simulink library "MBDS_Subsystems"  (R2018b)
settings: Solver=ode45  StartTime=0.0  StopTime=10.0  RelTol=1e-3
libraries: KIBES_Signal x1429, MBDS_Modules x44, simulink x2
(part 4 of 15)

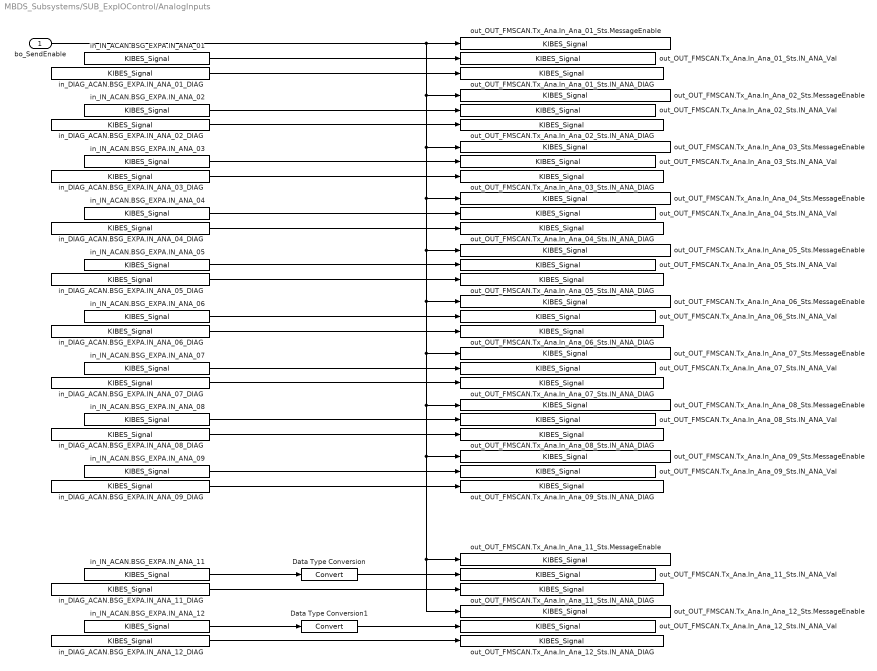
== system MBDS_Subsystems/SUB_ExpIOControl/AnalogInputs ==
  bo_SendEnable : Inport
  Data Type Conversion : DataTypeConversion  InitFcn=|  SaturateOnIntegerOverflow=on
      | try
      |    MBDS_BlockCallback('Update', gcb);
      | end
      settings: AttributesFormatString=Saturate: %<SaturateOnIntegerOverflow>
  Data Type Conversion1 : DataTypeConversion  InitFcn=|  SaturateOnIntegerOverflow=on
      | try
      |    MBDS_BlockCallback('Update', gcb);
      | end
      settings: AttributesFormatString=Saturate: %<SaturateOnIntegerOverflow>
  in_DIAG_ACAN.BSG_EXPA.IN_ANA_01_DIAG : KIBES_Signal/KIBES_Signal  MBDS_LibraryBlock=on  DatabaseKey=815  SignalName=DIAG_ACAN.BSG_EXPA.IN_ANA_01_DIAG  SymbolName=DIAG_ACAN_BSG_EXPA_IN_ANA_01_DIAG_000815  DataType=uint16  Init=1  Slope=1  Bias=0  DataSize=1  fpDataType=uint16  BlockIOType=Inport  DeviceType=0
  in_DIAG_ACAN.BSG_EXPA.IN_ANA_02_DIAG : KIBES_Signal/KIBES_Signal  MBDS_LibraryBlock=on  DatabaseKey=819  SignalName=DIAG_ACAN.BSG_EXPA.IN_ANA_02_DIAG  SymbolName=DIAG_ACAN_BSG_EXPA_IN_ANA_02_DIAG_000819  DataType=uint16  Init=1  Slope=1  Bias=0  DataSize=1  fpDataType=uint16  BlockIOType=Inport  DeviceType=0
  in_DIAG_ACAN.BSG_EXPA.IN_ANA_03_DIAG : KIBES_Signal/KIBES_Signal  MBDS_LibraryBlock=on  DatabaseKey=822  SignalName=DIAG_ACAN.BSG_EXPA.IN_ANA_03_DIAG  SymbolName=DIAG_ACAN_BSG_EXPA_IN_ANA_03_DIAG_000822  DataType=uint16  Init=1  Slope=1  Bias=0  DataSize=1  fpDataType=uint16  BlockIOType=Inport  DeviceType=0
  in_DIAG_ACAN.BSG_EXPA.IN_ANA_04_DIAG : KIBES_Signal/KIBES_Signal  MBDS_LibraryBlock=on  DatabaseKey=824  SignalName=DIAG_ACAN.BSG_EXPA.IN_ANA_04_DIAG  SymbolName=DIAG_ACAN_BSG_EXPA_IN_ANA_04_DIAG_000824  DataType=uint16  Init=1  Slope=1  Bias=0  DataSize=1  fpDataType=uint16  BlockIOType=Inport  DeviceType=0
  in_DIAG_ACAN.BSG_EXPA.IN_ANA_05_DIAG : KIBES_Signal/KIBES_Signal  MBDS_LibraryBlock=on  DatabaseKey=826  SignalName=DIAG_ACAN.BSG_EXPA.IN_ANA_05_DIAG  SymbolName=DIAG_ACAN_BSG_EXPA_IN_ANA_05_DIAG_000826  DataType=uint16  Init=1  Slope=1  Bias=0  DataSize=1  fpDataType=uint16  BlockIOType=Inport  DeviceType=0
  in_DIAG_ACAN.BSG_EXPA.IN_ANA_06_DIAG : KIBES_Signal/KIBES_Signal  MBDS_LibraryBlock=on  DatabaseKey=828  SignalName=DIAG_ACAN.BSG_EXPA.IN_ANA_06_DIAG  SymbolName=DIAG_ACAN_BSG_EXPA_IN_ANA_06_DIAG_000828  DataType=uint16  Init=1  Slope=1  Bias=0  DataSize=1  fpDataType=uint16  BlockIOType=Inport  DeviceType=0
  in_DIAG_ACAN.BSG_EXPA.IN_ANA_07_DIAG : KIBES_Signal/KIBES_Signal  MBDS_LibraryBlock=on  DatabaseKey=803  SignalName=DIAG_ACAN.BSG_EXPA.IN_ANA_07_DIAG  SymbolName=DIAG_ACAN_BSG_EXPA_IN_ANA_07_DIAG_000803  DataType=uint16  Init=1  Slope=1  Bias=0  DataSize=1  fpDataType=uint16  BlockIOType=Inport  DeviceType=0
  in_DIAG_ACAN.BSG_EXPA.IN_ANA_08_DIAG : KIBES_Signal/KIBES_Signal  MBDS_LibraryBlock=on  DatabaseKey=805  SignalName=DIAG_ACAN.BSG_EXPA.IN_ANA_08_DIAG  SymbolName=DIAG_ACAN_BSG_EXPA_IN_ANA_08_DIAG_000805  DataType=uint16  Init=1  Slope=1  Bias=0  DataSize=1  fpDataType=uint16  BlockIOType=Inport  DeviceType=0
  in_DIAG_ACAN.BSG_EXPA.IN_ANA_09_DIAG : KIBES_Signal/KIBES_Signal  MBDS_LibraryBlock=on  DatabaseKey=807  SignalName=DIAG_ACAN.BSG_EXPA.IN_ANA_09_DIAG  SymbolName=DIAG_ACAN_BSG_EXPA_IN_ANA_09_DIAG_000807  DataType=uint16  Init=1  Slope=1  Bias=0  DataSize=1  fpDataType=uint16  BlockIOType=Inport  DeviceType=0
  in_DIAG_ACAN.BSG_EXPA.IN_ANA_11_DIAG : KIBES_Signal/KIBES_Signal  MBDS_LibraryBlock=on  DatabaseKey=812  SignalName=DIAG_ACAN.BSG_EXPA.IN_ANA_11_DIAG  SymbolName=DIAG_ACAN_BSG_EXPA_IN_ANA_11_DIAG_000812  DataType=uint16  Init=1  Slope=1  Bias=0  DataSize=1  fpDataType=uint16  BlockIOType=Inport  DeviceType=0
  in_DIAG_ACAN.BSG_EXPA.IN_ANA_12_DIAG : KIBES_Signal/KIBES_Signal  MBDS_LibraryBlock=on  DatabaseKey=818  SignalName=DIAG_ACAN.BSG_EXPA.IN_ANA_12_DIAG  SymbolName=DIAG_ACAN_BSG_EXPA_IN_ANA_12_DIAG_000818  DataType=uint16  Init=1  Slope=1  Bias=0  DataSize=1  fpDataType=uint16  BlockIOType=Inport  DeviceType=0
  in_IN_ACAN.BSG_EXPA.IN_ANA_01 : KIBES_Signal/KIBES_Signal  MBDS_LibraryBlock=on  DatabaseKey=821  SignalName=IN_ACAN.BSG_EXPA.IN_ANA_01  SymbolName=IN_ACAN_BSG_EXPA_IN_ANA_01_000821  DataType=uint32  Init=0  Slope=1  Bias=0  DataSize=1  fpDataType=uint32  BlockIOType=Inport  DeviceType=0
  in_IN_ACAN.BSG_EXPA.IN_ANA_02 : KIBES_Signal/KIBES_Signal  MBDS_LibraryBlock=on  DatabaseKey=817  SignalName=IN_ACAN.BSG_EXPA.IN_ANA_02  SymbolName=IN_ACAN_BSG_EXPA_IN_ANA_02_000817  DataType=uint32  Init=0  Slope=1  Bias=0  DataSize=1  fpDataType=uint32  BlockIOType=Inport  DeviceType=0
  in_IN_ACAN.BSG_EXPA.IN_ANA_03 : KIBES_Signal/KIBES_Signal  MBDS_LibraryBlock=on  DatabaseKey=820  SignalName=IN_ACAN.BSG_EXPA.IN_ANA_03  SymbolName=IN_ACAN_BSG_EXPA_IN_ANA_03_000820  DataType=uint32  Init=0  Slope=1  Bias=0  DataSize=1  fpDataType=uint32  BlockIOType=Inport  DeviceType=0
  in_IN_ACAN.BSG_EXPA.IN_ANA_04 : KIBES_Signal/KIBES_Signal  MBDS_LibraryBlock=on  DatabaseKey=823  SignalName=IN_ACAN.BSG_EXPA.IN_ANA_04  SymbolName=IN_ACAN_BSG_EXPA_IN_ANA_04_000823  DataType=uint32  Init=0  Slope=1  Bias=0  DataSize=1  fpDataType=uint32  BlockIOType=Inport  DeviceType=0
  in_IN_ACAN.BSG_EXPA.IN_ANA_05 : KIBES_Signal/KIBES_Signal  MBDS_LibraryBlock=on  DatabaseKey=825  SignalName=IN_ACAN.BSG_EXPA.IN_ANA_05  SymbolName=IN_ACAN_BSG_EXPA_IN_ANA_05_000825  DataType=uint32  Init=0  Slope=1  Bias=0  DataSize=1  fpDataType=uint32  BlockIOType=Inport  DeviceType=0
  in_IN_ACAN.BSG_EXPA.IN_ANA_06 : KIBES_Signal/KIBES_Signal  MBDS_LibraryBlock=on  DatabaseKey=827  SignalName=IN_ACAN.BSG_EXPA.IN_ANA_06  SymbolName=IN_ACAN_BSG_EXPA_IN_ANA_06_000827  DataType=uint32  Init=0  Slope=1  Bias=0  DataSize=1  fpDataType=uint32  BlockIOType=Inport  DeviceType=0
  in_IN_ACAN.BSG_EXPA.IN_ANA_07 : KIBES_Signal/KIBES_Signal  MBDS_LibraryBlock=on  DatabaseKey=816  SignalName=IN_ACAN.BSG_EXPA.IN_ANA_07  SymbolName=IN_ACAN_BSG_EXPA_IN_ANA_07_000816  DataType=uint32  Init=0  Slope=1  Bias=0  DataSize=1  fpDataType=uint32  BlockIOType=Inport  DeviceType=0
  in_IN_ACAN.BSG_EXPA.IN_ANA_08 : KIBES_Signal/KIBES_Signal  MBDS_LibraryBlock=on  DatabaseKey=804  SignalName=IN_ACAN.BSG_EXPA.IN_ANA_08  SymbolName=IN_ACAN_BSG_EXPA_IN_ANA_08_000804  DataType=uint32  Init=0  Slope=1  Bias=0  DataSize=1  fpDataType=uint32  BlockIOType=Inport  DeviceType=0
  in_IN_ACAN.BSG_EXPA.IN_ANA_09 : KIBES_Signal/KIBES_Signal  MBDS_LibraryBlock=on  DatabaseKey=806  SignalName=IN_ACAN.BSG_EXPA.IN_ANA_09  SymbolName=IN_ACAN_BSG_EXPA_IN_ANA_09_000806  DataType=uint32  Init=0  Slope=1  Bias=0  DataSize=1  fpDataType=uint32  BlockIOType=Inport  DeviceType=0
  in_IN_ACAN.BSG_EXPA.IN_ANA_11 : KIBES_Signal/KIBES_Signal  MBDS_LibraryBlock=on  DatabaseKey=814  SignalName=IN_ACAN.BSG_EXPA.IN_ANA_11  SymbolName=IN_ACAN_BSG_EXPA_IN_ANA_11_000814  DataType=uint16  Init=0  Slope=1  Bias=0  DataSize=1  fpDataType=uint16  BlockIOType=Inport  DeviceType=0
  in_IN_ACAN.BSG_EXPA.IN_ANA_12 : KIBES_Signal/KIBES_Signal  MBDS_LibraryBlock=on  DatabaseKey=811  SignalName=IN_ACAN.BSG_EXPA.IN_ANA_12  SymbolName=IN_ACAN_BSG_EXPA_IN_ANA_12_000811  DataType=uint16  Init=0  Slope=1  Bias=0  DataSize=1  fpDataType=uint16  BlockIOType=Inport  DeviceType=0
  out_OUT_FMSCAN.Tx_Ana.In_Ana_01_Sts.IN_ANA_DIAG : KIBES_Signal/KIBES_Signal  MBDS_LibraryBlock=on  DatabaseKey=2579  SignalName=OUT_FMSCAN.Tx_Ana.In_Ana_01_Sts.IN_ANA_DIAG  SymbolName=OUT_FMSCAN_Tx_Ana_In_Ana_01_Sts_IN_ANA_DIAG_002579  DataType=uint16  Init=0  Slope=1  Bias=0  DataSize=1  fpDataType=uint16  BlockIOType=Outport  DeviceType=0
  out_OUT_FMSCAN.Tx_Ana.In_Ana_01_Sts.IN_ANA_Val : KIBES_Signal/KIBES_Signal  MBDS_LibraryBlock=on  DatabaseKey=2580  SignalName=OUT_FMSCAN.Tx_Ana.In_Ana_01_Sts.IN_ANA_Val  SymbolName=OUT_FMSCAN_Tx_Ana_In_Ana_01_Sts_IN_ANA_Val_002580  DataType=uint32  Init=0  Slope=1  Bias=0  DataSize=1  fpDataType=uint32  BlockIOType=Outport  DeviceType=0
  out_OUT_FMSCAN.Tx_Ana.In_Ana_01_Sts.MessageEnable : KIBES_Signal/KIBES_Signal  MBDS_LibraryBlock=on  DatabaseKey=2603  SignalName=OUT_FMSCAN.Tx_Ana.In_Ana_01_Sts.MessageEnable  SymbolName=OUT_FMSCAN_Tx_Ana_In_Ana_01_Sts_MessageEnable_002603  DataType=boolean  Init=0  Slope=1  Bias=0  DataSize=1  fpDataType=boolean  BlockIOType=Outport  DeviceType=0
  out_OUT_FMSCAN.Tx_Ana.In_Ana_02_Sts.IN_ANA_DIAG : KIBES_Signal/KIBES_Signal  MBDS_LibraryBlock=on  DatabaseKey=2581  SignalName=OUT_FMSCAN.Tx_Ana.In_Ana_02_Sts.IN_ANA_DIAG  SymbolName=OUT_FMSCAN_Tx_Ana_In_Ana_02_Sts_IN_ANA_DIAG_002581  DataType=uint16  Init=0  Slope=1  Bias=0  DataSize=1  fpDataType=uint16  BlockIOType=Outport  DeviceType=0
  out_OUT_FMSCAN.Tx_Ana.In_Ana_02_Sts.IN_ANA_Val : KIBES_Signal/KIBES_Signal  MBDS_LibraryBlock=on  DatabaseKey=2582  SignalName=OUT_FMSCAN.Tx_Ana.In_Ana_02_Sts.IN_ANA_Val  SymbolName=OUT_FMSCAN_Tx_Ana_In_Ana_02_Sts_IN_ANA_Val_002582  DataType=uint32  Init=0  Slope=1  Bias=0  DataSize=1  fpDataType=uint32  BlockIOType=Outport  DeviceType=0
  out_OUT_FMSCAN.Tx_Ana.In_Ana_02_Sts.MessageEnable : KIBES_Signal/KIBES_Signal  MBDS_LibraryBlock=on  DatabaseKey=2604  SignalName=OUT_FMSCAN.Tx_Ana.In_Ana_02_Sts.MessageEnable  SymbolName=OUT_FMSCAN_Tx_Ana_In_Ana_02_Sts_MessageEnable_002604  DataType=boolean  Init=0  Slope=1  Bias=0  DataSize=1  fpDataType=boolean  BlockIOType=Outport  DeviceType=0
  out_OUT_FMSCAN.Tx_Ana.In_Ana_03_Sts.IN_ANA_DIAG : KIBES_Signal/KIBES_Signal  MBDS_LibraryBlock=on  DatabaseKey=2583  SignalName=OUT_FMSCAN.Tx_Ana.In_Ana_03_Sts.IN_ANA_DIAG  SymbolName=OUT_FMSCAN_Tx_Ana_In_Ana_03_Sts_IN_ANA_DIAG_002583  DataType=uint16  Init=0  Slope=1  Bias=0  DataSize=1  fpDataType=uint16  BlockIOType=Outport  DeviceType=0
  out_OUT_FMSCAN.Tx_Ana.In_Ana_03_Sts.IN_ANA_Val : KIBES_Signal/KIBES_Signal  MBDS_LibraryBlock=on  DatabaseKey=2584  SignalName=OUT_FMSCAN.Tx_Ana.In_Ana_03_Sts.IN_ANA_Val  SymbolName=OUT_FMSCAN_Tx_Ana_In_Ana_03_Sts_IN_ANA_Val_002584  DataType=uint32  Init=0  Slope=1  Bias=0  DataSize=1  fpDataType=uint32  BlockIOType=Outport  DeviceType=0
  out_OUT_FMSCAN.Tx_Ana.In_Ana_03_Sts.MessageEnable : KIBES_Signal/KIBES_Signal  MBDS_LibraryBlock=on  DatabaseKey=2605  SignalName=OUT_FMSCAN.Tx_Ana.In_Ana_03_Sts.MessageEnable  SymbolName=OUT_FMSCAN_Tx_Ana_In_Ana_03_Sts_MessageEnable_002605  DataType=boolean  Init=0  Slope=1  Bias=0  DataSize=1  fpDataType=boolean  BlockIOType=Outport  DeviceType=0
  out_OUT_FMSCAN.Tx_Ana.In_Ana_04_Sts.IN_ANA_DIAG : KIBES_Signal/KIBES_Signal  MBDS_LibraryBlock=on  DatabaseKey=2585  SignalName=OUT_FMSCAN.Tx_Ana.In_Ana_04_Sts.IN_ANA_DIAG  SymbolName=OUT_FMSCAN_Tx_Ana_In_Ana_04_Sts_IN_ANA_DIAG_002585  DataType=uint16  Init=0  Slope=1  Bias=0  DataSize=1  fpDataType=uint16  BlockIOType=Outport  DeviceType=0
  out_OUT_FMSCAN.Tx_Ana.In_Ana_04_Sts.IN_ANA_Val : KIBES_Signal/KIBES_Signal  MBDS_LibraryBlock=on  DatabaseKey=2586  SignalName=OUT_FMSCAN.Tx_Ana.In_Ana_04_Sts.IN_ANA_Val  SymbolName=OUT_FMSCAN_Tx_Ana_In_Ana_04_Sts_IN_ANA_Val_002586  DataType=uint32  Init=0  Slope=1  Bias=0  DataSize=1  fpDataType=uint32  BlockIOType=Outport  DeviceType=0
  out_OUT_FMSCAN.Tx_Ana.In_Ana_04_Sts.MessageEnable : KIBES_Signal/KIBES_Signal  MBDS_LibraryBlock=on  DatabaseKey=2606  SignalName=OUT_FMSCAN.Tx_Ana.In_Ana_04_Sts.MessageEnable  SymbolName=OUT_FMSCAN_Tx_Ana_In_Ana_04_Sts_MessageEnable_002606  DataType=boolean  Init=0  Slope=1  Bias=0  DataSize=1  fpDataType=boolean  BlockIOType=Outport  DeviceType=0
  out_OUT_FMSCAN.Tx_Ana.In_Ana_05_Sts.IN_ANA_DIAG : KIBES_Signal/KIBES_Signal  MBDS_LibraryBlock=on  DatabaseKey=2587  SignalName=OUT_FMSCAN.Tx_Ana.In_Ana_05_Sts.IN_ANA_DIAG  SymbolName=OUT_FMSCAN_Tx_Ana_In_Ana_05_Sts_IN_ANA_DIAG_002587  DataType=uint16  Init=0  Slope=1  Bias=0  DataSize=1  fpDataType=uint16  BlockIOType=Outport  DeviceType=0
  out_OUT_FMSCAN.Tx_Ana.In_Ana_05_Sts.IN_ANA_Val : KIBES_Signal/KIBES_Signal  MBDS_LibraryBlock=on  DatabaseKey=2588  SignalName=OUT_FMSCAN.Tx_Ana.In_Ana_05_Sts.IN_ANA_Val  SymbolName=OUT_FMSCAN_Tx_Ana_In_Ana_05_Sts_IN_ANA_Val_002588  DataType=uint32  Init=0  Slope=1  Bias=0  DataSize=1  fpDataType=uint32  BlockIOType=Outport  DeviceType=0
  out_OUT_FMSCAN.Tx_Ana.In_Ana_05_Sts.MessageEnable : KIBES_Signal/KIBES_Signal  MBDS_LibraryBlock=on  DatabaseKey=2607  SignalName=OUT_FMSCAN.Tx_Ana.In_Ana_05_Sts.MessageEnable  SymbolName=OUT_FMSCAN_Tx_Ana_In_Ana_05_Sts_MessageEnable_002607  DataType=boolean  Init=0  Slope=1  Bias=0  DataSize=1  fpDataType=boolean  BlockIOType=Outport  DeviceType=0
  out_OUT_FMSCAN.Tx_Ana.In_Ana_06_Sts.IN_ANA_DIAG : KIBES_Signal/KIBES_Signal  MBDS_LibraryBlock=on  DatabaseKey=2589  SignalName=OUT_FMSCAN.Tx_Ana.In_Ana_06_Sts.IN_ANA_DIAG  SymbolName=OUT_FMSCAN_Tx_Ana_In_Ana_06_Sts_IN_ANA_DIAG_002589  DataType=uint16  Init=0  Slope=1  Bias=0  DataSize=1  fpDataType=uint16  BlockIOType=Outport  DeviceType=0
  out_OUT_FMSCAN.Tx_Ana.In_Ana_06_Sts.IN_ANA_Val : KIBES_Signal/KIBES_Signal  MBDS_LibraryBlock=on  DatabaseKey=2590  SignalName=OUT_FMSCAN.Tx_Ana.In_Ana_06_Sts.IN_ANA_Val  SymbolName=OUT_FMSCAN_Tx_Ana_In_Ana_06_Sts_IN_ANA_Val_002590  DataType=uint32  Init=0  Slope=1  Bias=0  DataSize=1  fpDataType=uint32  BlockIOType=Outport  DeviceType=0
  out_OUT_FMSCAN.Tx_Ana.In_Ana_06_Sts.MessageEnable : KIBES_Signal/KIBES_Signal  MBDS_LibraryBlock=on  DatabaseKey=2608  SignalName=OUT_FMSCAN.Tx_Ana.In_Ana_06_Sts.MessageEnable  SymbolName=OUT_FMSCAN_Tx_Ana_In_Ana_06_Sts_MessageEnable_002608  DataType=boolean  Init=0  Slope=1  Bias=0  DataSize=1  fpDataType=boolean  BlockIOType=Outport  DeviceType=0
  out_OUT_FMSCAN.Tx_Ana.In_Ana_07_Sts.IN_ANA_DIAG : KIBES_Signal/KIBES_Signal  MBDS_LibraryBlock=on  DatabaseKey=2591  SignalName=OUT_FMSCAN.Tx_Ana.In_Ana_07_Sts.IN_ANA_DIAG  SymbolName=OUT_FMSCAN_Tx_Ana_In_Ana_07_Sts_IN_ANA_DIAG_002591  DataType=uint16  Init=0  Slope=1  Bias=0  DataSize=1  fpDataType=uint16  BlockIOType=Outport  DeviceType=0
  out_OUT_FMSCAN.Tx_Ana.In_Ana_07_Sts.IN_ANA_Val : KIBES_Signal/KIBES_Signal  MBDS_LibraryBlock=on  DatabaseKey=2592  SignalName=OUT_FMSCAN.Tx_Ana.In_Ana_07_Sts.IN_ANA_Val  SymbolName=OUT_FMSCAN_Tx_Ana_In_Ana_07_Sts_IN_ANA_Val_002592  DataType=uint32  Init=0  Slope=1  Bias=0  DataSize=1  fpDataType=uint32  BlockIOType=Outport  DeviceType=0
  out_OUT_FMSCAN.Tx_Ana.In_Ana_07_Sts.MessageEnable : KIBES_Signal/KIBES_Signal  MBDS_LibraryBlock=on  DatabaseKey=2609  SignalName=OUT_FMSCAN.Tx_Ana.In_Ana_07_Sts.MessageEnable  SymbolName=OUT_FMSCAN_Tx_Ana_In_Ana_07_Sts_MessageEnable_002609  DataType=boolean  Init=0  Slope=1  Bias=0  DataSize=1  fpDataType=boolean  BlockIOType=Outport  DeviceType=0
  out_OUT_FMSCAN.Tx_Ana.In_Ana_08_Sts.IN_ANA_DIAG : KIBES_Signal/KIBES_Signal  MBDS_LibraryBlock=on  DatabaseKey=2593  SignalName=OUT_FMSCAN.Tx_Ana.In_Ana_08_Sts.IN_ANA_DIAG  SymbolName=OUT_FMSCAN_Tx_Ana_In_Ana_08_Sts_IN_ANA_DIAG_002593  DataType=uint16  Init=0  Slope=1  Bias=0  DataSize=1  fpDataType=uint16  BlockIOType=Outport  DeviceType=0
  out_OUT_FMSCAN.Tx_Ana.In_Ana_08_Sts.IN_ANA_Val : KIBES_Signal/KIBES_Signal  MBDS_LibraryBlock=on  DatabaseKey=2594  SignalName=OUT_FMSCAN.Tx_Ana.In_Ana_08_Sts.IN_ANA_Val  SymbolName=OUT_FMSCAN_Tx_Ana_In_Ana_08_Sts_IN_ANA_Val_002594  DataType=uint32  Init=0  Slope=1  Bias=0  DataSize=1  fpDataType=uint32  BlockIOType=Outport  DeviceType=0
  out_OUT_FMSCAN.Tx_Ana.In_Ana_08_Sts.MessageEnable : KIBES_Signal/KIBES_Signal  MBDS_LibraryBlock=on  DatabaseKey=2610  SignalName=OUT_FMSCAN.Tx_Ana.In_Ana_08_Sts.MessageEnable  SymbolName=OUT_FMSCAN_Tx_Ana_In_Ana_08_Sts_MessageEnable_002610  DataType=boolean  Init=0  Slope=1  Bias=0  DataSize=1  fpDataType=boolean  BlockIOType=Outport  DeviceType=0
  out_OUT_FMSCAN.Tx_Ana.In_Ana_09_Sts.IN_ANA_DIAG : KIBES_Signal/KIBES_Signal  MBDS_LibraryBlock=on  DatabaseKey=2595  SignalName=OUT_FMSCAN.Tx_Ana.In_Ana_09_Sts.IN_ANA_DIAG  SymbolName=OUT_FMSCAN_Tx_Ana_In_Ana_09_Sts_IN_ANA_DIAG_002595  DataType=uint16  Init=0  Slope=1  Bias=0  DataSize=1  fpDataType=uint16  BlockIOType=Outport  DeviceType=0
  out_OUT_FMSCAN.Tx_Ana.In_Ana_09_Sts.IN_ANA_Val : KIBES_Signal/KIBES_Signal  MBDS_LibraryBlock=on  DatabaseKey=2596  SignalName=OUT_FMSCAN.Tx_Ana.In_Ana_09_Sts.IN_ANA_Val  SymbolName=OUT_FMSCAN_Tx_Ana_In_Ana_09_Sts_IN_ANA_Val_002596  DataType=uint32  Init=0  Slope=1  Bias=0  DataSize=1  fpDataType=uint32  BlockIOType=Outport  DeviceType=0
  out_OUT_FMSCAN.Tx_Ana.In_Ana_09_Sts.MessageEnable : KIBES_Signal/KIBES_Signal  MBDS_LibraryBlock=on  DatabaseKey=2611  SignalName=OUT_FMSCAN.Tx_Ana.In_Ana_09_Sts.MessageEnable  SymbolName=OUT_FMSCAN_Tx_Ana_In_Ana_09_Sts_MessageEnable_002611  DataType=boolean  Init=0  Slope=1  Bias=0  DataSize=1  fpDataType=boolean  BlockIOType=Outport  DeviceType=0
  out_OUT_FMSCAN.Tx_Ana.In_Ana_11_Sts.IN_ANA_DIAG : KIBES_Signal/KIBES_Signal  MBDS_LibraryBlock=on  DatabaseKey=2599  SignalName=OUT_FMSCAN.Tx_Ana.In_Ana_11_Sts.IN_ANA_DIAG  SymbolName=OUT_FMSCAN_Tx_Ana_In_Ana_11_Sts_IN_ANA_DIAG_002599  DataType=uint16  Init=0  Slope=1  Bias=0  DataSize=1  fpDataType=uint16  BlockIOType=Outport  DeviceType=0
  out_OUT_FMSCAN.Tx_Ana.In_Ana_11_Sts.IN_ANA_Val : KIBES_Signal/KIBES_Signal  MBDS_LibraryBlock=on  DatabaseKey=2600  SignalName=OUT_FMSCAN.Tx_Ana.In_Ana_11_Sts.IN_ANA_Val  SymbolName=OUT_FMSCAN_Tx_Ana_In_Ana_11_Sts_IN_ANA_Val_002600  DataType=uint32  Init=0  Slope=1  Bias=0  DataSize=1  fpDataType=uint32  BlockIOType=Outport  DeviceType=0
  out_OUT_FMSCAN.Tx_Ana.In_Ana_11_Sts.MessageEnable : KIBES_Signal/KIBES_Signal  MBDS_LibraryBlock=on  DatabaseKey=2613  SignalName=OUT_FMSCAN.Tx_Ana.In_Ana_11_Sts.MessageEnable  SymbolName=OUT_FMSCAN_Tx_Ana_In_Ana_11_Sts_MessageEnable_002613  DataType=boolean  Init=0  Slope=1  Bias=0  DataSize=1  fpDataType=boolean  BlockIOType=Outport  DeviceType=0
  out_OUT_FMSCAN.Tx_Ana.In_Ana_12_Sts.IN_ANA_DIAG : KIBES_Signal/KIBES_Signal  MBDS_LibraryBlock=on  DatabaseKey=2601  SignalName=OUT_FMSCAN.Tx_Ana.In_Ana_12_Sts.IN_ANA_DIAG  SymbolName=OUT_FMSCAN_Tx_Ana_In_Ana_12_Sts_IN_ANA_DIAG_002601  DataType=uint16  Init=0  Slope=1  Bias=0  DataSize=1  fpDataType=uint16  BlockIOType=Outport  DeviceType=0
  out_OUT_FMSCAN.Tx_Ana.In_Ana_12_Sts.IN_ANA_Val : KIBES_Signal/KIBES_Signal  MBDS_LibraryBlock=on  DatabaseKey=2602  SignalName=OUT_FMSCAN.Tx_Ana.In_Ana_12_Sts.IN_ANA_Val  SymbolName=OUT_FMSCAN_Tx_Ana_In_Ana_12_Sts_IN_ANA_Val_002602  DataType=uint32  Init=0  Slope=1  Bias=0  DataSize=1  fpDataType=uint32  BlockIOType=Outport  DeviceType=0
  out_OUT_FMSCAN.Tx_Ana.In_Ana_12_Sts.MessageEnable : KIBES_Signal/KIBES_Signal  MBDS_LibraryBlock=on  DatabaseKey=2614  SignalName=OUT_FMSCAN.Tx_Ana.In_Ana_12_Sts.MessageEnable  SymbolName=OUT_FMSCAN_Tx_Ana_In_Ana_12_Sts_MessageEnable_002614  DataType=boolean  Init=0  Slope=1  Bias=0  DataSize=1  fpDataType=boolean  BlockIOType=Outport  DeviceType=0
  wires:
  Data Type Conversion1/1 -> out_OUT_FMSCAN.Tx_Ana.In_Ana_12_Sts.IN_ANA_Val/1
  Data Type Conversion/1 -> out_OUT_FMSCAN.Tx_Ana.In_Ana_11_Sts.IN_ANA_Val/1
  in_IN_ACAN.BSG_EXPA.IN_ANA_05/1 -> out_OUT_FMSCAN.Tx_Ana.In_Ana_05_Sts.IN_ANA_Val/1
  in_IN_ACAN.BSG_EXPA.IN_ANA_04/1 -> out_OUT_FMSCAN.Tx_Ana.In_Ana_04_Sts.IN_ANA_Val/1
  in_DIAG_ACAN.BSG_EXPA.IN_ANA_03_DIAG/1 -> out_OUT_FMSCAN.Tx_Ana.In_Ana_03_Sts.IN_ANA_DIAG/1
  in_DIAG_ACAN.BSG_EXPA.IN_ANA_04_DIAG/1 -> out_OUT_FMSCAN.Tx_Ana.In_Ana_04_Sts.IN_ANA_DIAG/1
  in_DIAG_ACAN.BSG_EXPA.IN_ANA_11_DIAG/1 -> out_OUT_FMSCAN.Tx_Ana.In_Ana_11_Sts.IN_ANA_DIAG/1
  in_DIAG_ACAN.BSG_EXPA.IN_ANA_12_DIAG/1 -> out_OUT_FMSCAN.Tx_Ana.In_Ana_12_Sts.IN_ANA_DIAG/1
  in_IN_ACAN.BSG_EXPA.IN_ANA_07/1 -> out_OUT_FMSCAN.Tx_Ana.In_Ana_07_Sts.IN_ANA_Val/1
  in_DIAG_ACAN.BSG_EXPA.IN_ANA_01_DIAG/1 -> out_OUT_FMSCAN.Tx_Ana.In_Ana_01_Sts.IN_ANA_DIAG/1
  in_IN_ACAN.BSG_EXPA.IN_ANA_11/1 -> Data Type Conversion/1
  in_DIAG_ACAN.BSG_EXPA.IN_ANA_05_DIAG/1 -> out_OUT_FMSCAN.Tx_Ana.In_Ana_05_Sts.IN_ANA_DIAG/1
  in_IN_ACAN.BSG_EXPA.IN_ANA_06/1 -> out_OUT_FMSCAN.Tx_Ana.In_Ana_06_Sts.IN_ANA_Val/1
  in_IN_ACAN.BSG_EXPA.IN_ANA_03/1 -> out_OUT_FMSCAN.Tx_Ana.In_Ana_03_Sts.IN_ANA_Val/1
  in_DIAG_ACAN.BSG_EXPA.IN_ANA_07_DIAG/1 -> out_OUT_FMSCAN.Tx_Ana.In_Ana_07_Sts.IN_ANA_DIAG/1
  in_IN_ACAN.BSG_EXPA.IN_ANA_01/1 -> out_OUT_FMSCAN.Tx_Ana.In_Ana_01_Sts.IN_ANA_Val/1
  in_IN_ACAN.BSG_EXPA.IN_ANA_08/1 -> out_OUT_FMSCAN.Tx_Ana.In_Ana_08_Sts.IN_ANA_Val/1
  in_IN_ACAN.BSG_EXPA.IN_ANA_02/1 -> out_OUT_FMSCAN.Tx_Ana.In_Ana_02_Sts.IN_ANA_Val/1
  in_DIAG_ACAN.BSG_EXPA.IN_ANA_08_DIAG/1 -> out_OUT_FMSCAN.Tx_Ana.In_Ana_08_Sts.IN_ANA_DIAG/1
  in_DIAG_ACAN.BSG_EXPA.IN_ANA_02_DIAG/1 -> out_OUT_FMSCAN.Tx_Ana.In_Ana_02_Sts.IN_ANA_DIAG/1
  in_IN_ACAN.BSG_EXPA.IN_ANA_09/1 -> out_OUT_FMSCAN.Tx_Ana.In_Ana_09_Sts.IN_ANA_Val/1
  in_IN_ACAN.BSG_EXPA.IN_ANA_12/1 -> Data Type Conversion1/1
  in_DIAG_ACAN.BSG_EXPA.IN_ANA_06_DIAG/1 -> out_OUT_FMSCAN.Tx_Ana.In_Ana_06_Sts.IN_ANA_DIAG/1
  bo_SendEnable/1 -> out_OUT_FMSCAN.Tx_Ana.In_Ana_11_Sts.MessageEnable/1, out_OUT_FMSCAN.Tx_Ana.In_Ana_12_Sts.MessageEnable/1, out_OUT_FMSCAN.Tx_Ana.In_Ana_09_Sts.MessageEnable/1, out_OUT_FMSCAN.Tx_Ana.In_Ana_08_Sts.MessageEnable/1, out_OUT_FMSCAN.Tx_Ana.In_Ana_07_Sts.MessageEnable/1, out_OUT_FMSCAN.Tx_Ana.In_Ana_06_Sts.MessageEnable/1, out_OUT_FMSCAN.Tx_Ana.In_Ana_05_Sts.MessageEnable/1, out_OUT_FMSCAN.Tx_Ana.In_Ana_04_Sts.MessageEnable/1, out_OUT_FMSCAN.Tx_Ana.In_Ana_03_Sts.MessageEnable/1, out_OUT_FMSCAN.Tx_Ana.In_Ana_02_Sts.MessageEnable/1, out_OUT_FMSCAN.Tx_Ana.In_Ana_01_Sts.MessageEnable/1
  in_DIAG_ACAN.BSG_EXPA.IN_ANA_09_DIAG/1 -> out_OUT_FMSCAN.Tx_Ana.In_Ana_09_Sts.IN_ANA_DIAG/1
